simulink model "On_off_1_pumpstation"  (R2022b)
settings: Solver=VariableStepAuto  StartTime=0.0  StopTime=inf  RelTol=1e-3
libraries: modbusMatLib x24, realtime_pacer_lib x1
(part 1 of 2)
settings Model: Creator=pppc  LastModifiedBy=pppc
settings SolverCC: AlgebraicLoopSolver=TrustRegion
settings DebuggingCC: UnconnectedInputMsg=warning  UnconnectedOutputMsg=warning  UnconnectedLineMsg=warning  SFMachineParentedDataDiag=warning
settings ModelReferenceCC: EnableRefExpFcnMdlSchedulingChecks=on
settings RTWCC: DLArmComputeVersion=19.05

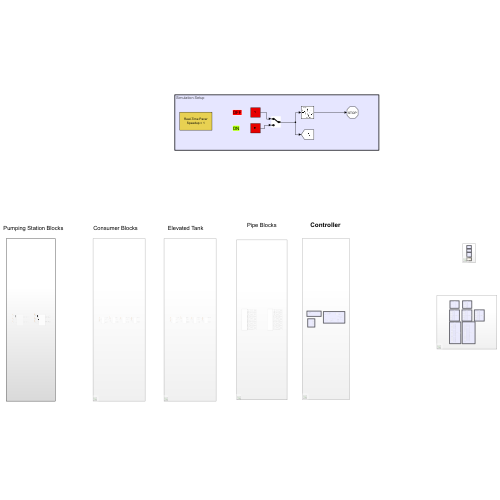
[thumbnail: Simulink's stored preview of the top-level diagram]
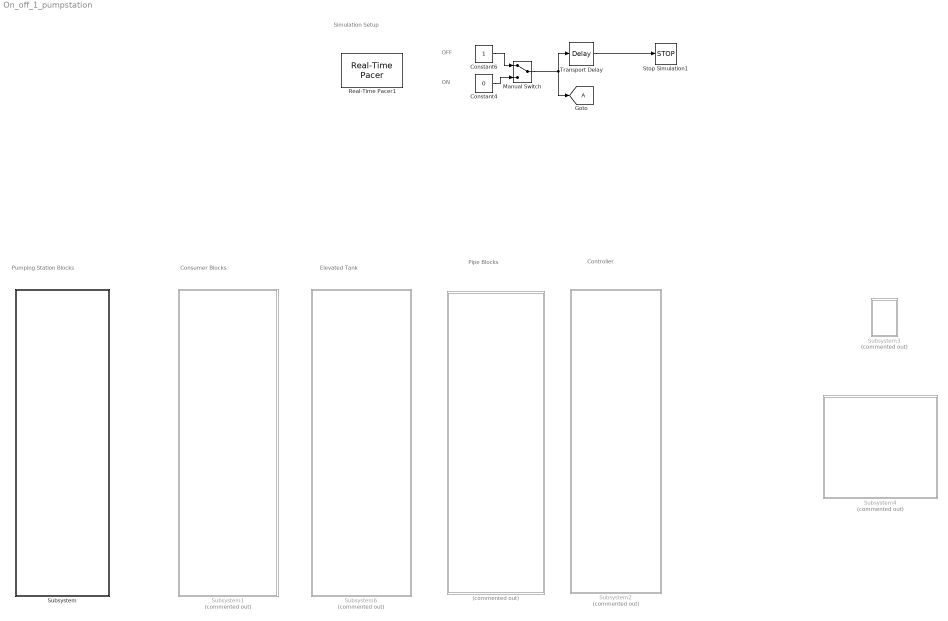
== system On_off_1_pumpstation ==
  note: Controller
  note: Pumping Station Blocks
  note: OFF
  note: ON
  note: Simulation Setup
  note: Consumer Blocks
  note: Pipe Blocks
  note: Elevated Tank
  " " : Subsystem  Commented=on
  Constant4 : Constant  Value=0
  Constant6 : Constant
  Goto : Goto  TagVisibility=global
  Manual Switch : ManualSwitch
  Real-Time Pacer1 : realtime_pacer_lib/Real-Time Pacer  simTimePerRealTime=1
  Stop Simulation1 : Stop
  Subsystem : Subsystem
  Subsystem1 : Subsystem  Commented=on
  Subsystem2 : Subsystem  Commented=on
  Subsystem3 : Subsystem  Commented=on
  Subsystem4 : Subsystem  Commented=on
  Subsystem6 : Subsystem  Commented=on
  Transport Delay : TransportDelay  DelayTime=2
  wires:
  Constant4/1 -> Manual Switch/2
  Transport Delay/1 -> Stop Simulation1/1
  Constant6/1 -> Manual Switch/1
  Manual Switch/1 -> Goto/1, Transport Delay/1

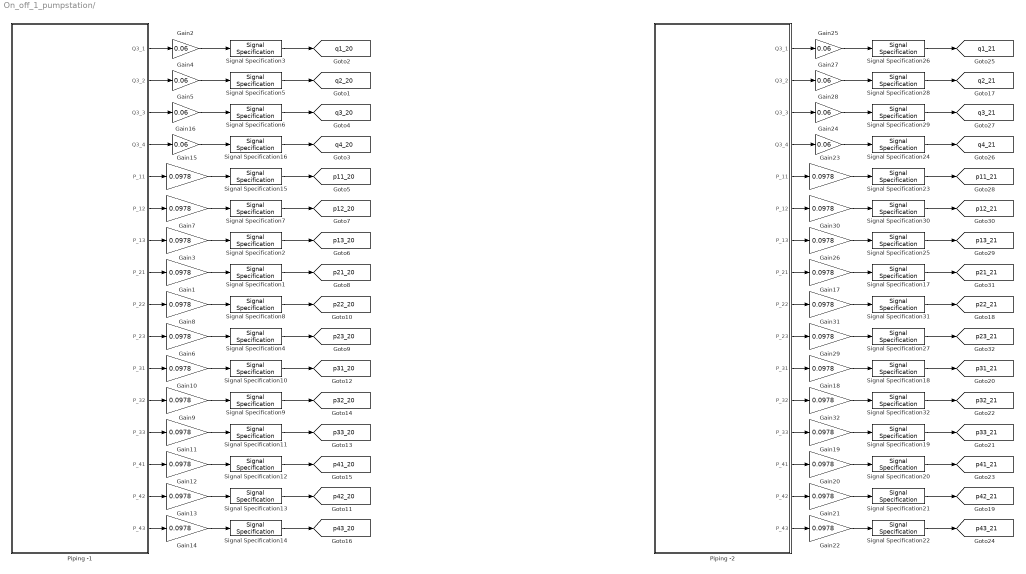
== system On_off_1_pumpstation/  ==
  Gain{1,3,6..15,17..23,26,29..32} (24 alike) : Gain  Gain=0.0978
  Gain{2,4..5,16,24..25,27..28} (8 alike) : Gain  Gain=0.06
  Piping -1 : Subsystem
  Piping -2 : Subsystem
  Signal Specification{1..2,4,7..15,17..23,25,27,30..32} (24 alike) : SignalSpecification  Unit=bar
  Signal Specification{3,5..6,16,24,26,28..29} (8 alike) : SignalSpecification  Unit=m^3/hr
  tag scope: p11_20=global, p11_21=global, p12_20=global, p12_21=global, p13_20=global, p13_21=global, p21_20=global, p21_21=global, p22_20=global, p22_21=global, p23_20=global, p23_21=global, p31_20=global, p31_21=global, p32_20=global, p32_21=global, p33_20=global, p33_21=global, p41_20=global, p41_21=global, p42_20=global, p42_21=global, p43_20=global, p43_21=global, q1_20=global, q1_21=global, q2_20=global, q2_21=global, q3_20=global, q3_21=global, q4_20=global, q4_21=global
  wires:
  Gain8/1 -> Signal Specification8/1
  Piping -1/6(P_12) -> Gain7/1
  Gain5/1 -> Signal Specification6/1
  Gain9/1 -> Signal Specification9/1
  Piping -1/12(P_32) -> Gain9/1
  Piping -1/9(P_22) -> Gain8/1
  Piping -1/3(Q3_3) -> Gain5/1
  Piping -1/2(Q3_2) -> Gain4/1
  Gain7/1 -> Signal Specification7/1
  Gain4/1 -> Signal Specification5/1
  Gain16/1 -> Signal Specification16/1
  Piping -1/4(Q3_4) -> Gain16/1
  Piping -1/1(Q3_1) -> Gain2/1
  Piping -1/8(P_21) -> Gain1/1
  Gain1/1 -> Signal Specification1/1
  Gain2/1 -> Signal Specification3/1
  Gain3/1 -> Signal Specification2/1
  Piping -1/7(P_13) -> Gain3/1
  Piping -1/10(P_23) -> Gain6/1
  Gain6/1 -> Signal Specification4/1
  Gain10/1 -> Signal Specification10/1
  Piping -1/11(P_31) -> Gain10/1
  Gain11/1 -> Signal Specification11/1
  Gain12/1 -> Signal Specification12/1
  Piping -1/13(P_33) -> Gain11/1
  Piping -1/14(P_41) -> Gain12/1
  Gain13/1 -> Signal Specification13/1
  Piping -1/15(P_42) -> Gain13/1
  Gain14/1 -> Signal Specification14/1
  Piping -1/16(P_43) -> Gain14/1
  Gain15/1 -> Signal Specification15/1
  Piping -1/5(P_11) -> Gain15/1
  Gain29/1 -> Signal Specification27/1
  Gain26/1 -> Signal Specification25/1
  Gain21/1 -> Signal Specification21/1
  Gain23/1 -> Signal Specification23/1
  Gain31/1 -> Signal Specification31/1
  Piping -2/15(P_42) -> Gain21/1
  Piping -2/5(P_11) -> Gain23/1
  Piping -2/16(P_43) -> Gain22/1
  Gain27/1 -> Signal Specification28/1
  Gain20/1 -> Signal Specification20/1
  Gain19/1 -> Signal Specification19/1
  Piping -2/14(P_41) -> Gain20/1
  Piping -2/13(P_33) -> Gain19/1
  Piping -2/12(P_32) -> Gain32/1
  Piping -2/6(P_12) -> Gain30/1
  Gain17/1 -> Signal Specification17/1
  Gain30/1 -> Signal Specification30/1
  Piping -2/3(Q3_3) -> Gain28/1
  Piping -2/7(P_13) -> Gain26/1
  Gain18/1 -> Signal Specification18/1
  Gain25/1 -> Signal Specification26/1
  Piping -2/4(Q3_4) -> Gain24/1
  Gain24/1 -> Signal Specification24/1
  Piping -2/8(P_21) -> Gain17/1
  Piping -2/1(Q3_1) -> Gain25/1
  Piping -2/11(P_31) -> Gain18/1
  Piping -2/9(P_22) -> Gain31/1
  Piping -2/10(P_23) -> Gain29/1
  Gain32/1 -> Signal Specification32/1
  Gain28/1 -> Signal Specification29/1
  Piping -2/2(Q3_2) -> Gain27/1
  Gain22/1 -> Signal Specification22/1
  Signal Specification3/1 -> [q1_20]
  Signal Specification5/1 -> [q2_20]
  Signal Specification6/1 -> [q3_20]
  Signal Specification16/1 -> [q4_20]
  Signal Specification2/1 -> [p13_20]
  Signal Specification15/1 -> [p11_20]
  Signal Specification7/1 -> [p12_20]
  Signal Specification8/1 -> [p22_20]
  Signal Specification4/1 -> [p23_20]
  Signal Specification1/1 -> [p21_20]
  Signal Specification13/1 -> [p42_20]
  Signal Specification12/1 -> [p41_20]
  Signal Specification14/1 -> [p43_20]
  Signal Specification9/1 -> [p32_20]
  Signal Specification11/1 -> [p33_20]
  Signal Specification10/1 -> [p31_20]
  Signal Specification32/1 -> [p32_21]
  Signal Specification26/1 -> [q1_21]
  Signal Specification21/1 -> [p42_21]
  Signal Specification19/1 -> [p33_21]
  Signal Specification20/1 -> [p41_21]
  Signal Specification18/1 -> [p31_21]
  Signal Specification27/1 -> [p23_21]
  Signal Specification31/1 -> [p22_21]
  Signal Specification24/1 -> [q4_21]
  Signal Specification30/1 -> [p12_21]
  Signal Specification23/1 -> [p11_21]
  Signal Specification28/1 -> [q2_21]
  Signal Specification29/1 -> [q3_21]
  Signal Specification17/1 -> [p21_21]
  Signal Specification22/1 -> [p43_21]
  Signal Specification25/1 -> [p13_21]

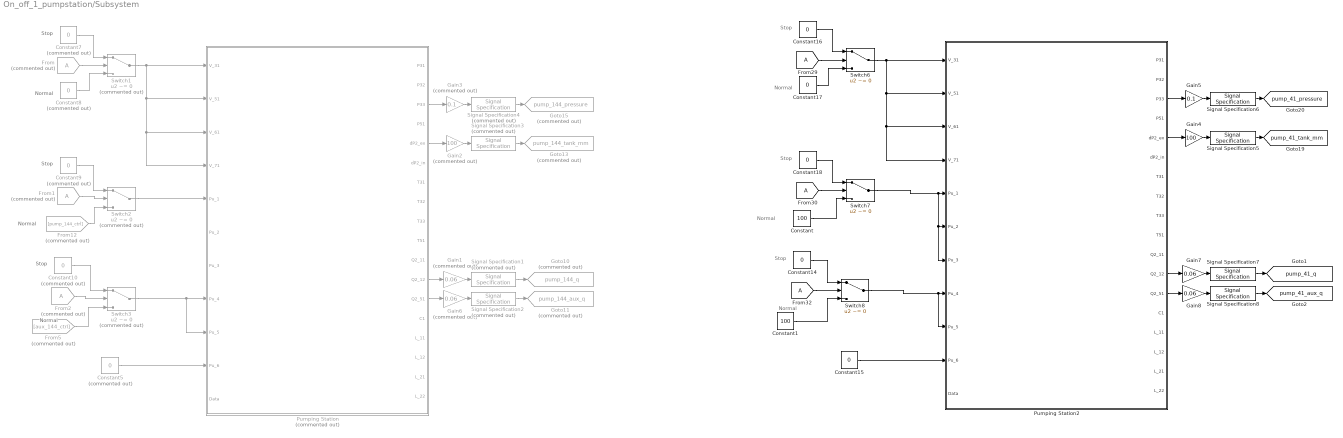
== system On_off_1_pumpstation/Subsystem ==
  note: Stop
  note: Normal
  note: Stop
  note: Normal
  note: Normal
  note: Stop
  note: Normal
  note: Stop
  note: Stop
  note: Normal
  note: Normal
  note: Stop
  Constant : Constant  Value=100
  Constant1 : Constant  Value=100
  Constant{5,7..10} (5 alike) : Constant  Commented=on  Value=0
  Constant{14..18} (5 alike) : Constant  Value=0
  From : From  Commented=on  TagVisibility=global
  From1 : From  Commented=on  TagVisibility=global
  From12 : From  Commented=on  GotoTag=pump_144_ctrl  TagVisibility=global
  From2 : From  Commented=on  TagVisibility=global
  From29 : From  TagVisibility=global
  From30 : From  TagVisibility=global
  From32 : From  TagVisibility=global
  From5 : From  Commented=on  GotoTag=aux_144_ctrl  TagVisibility=global
  Gain1 : Gain  Commented=on  Gain=0.06
  Gain2 : Gain  Commented=on  Gain=100
  Gain3 : Gain  Commented=on  Gain=0.1
  Gain4 : Gain  Gain=100
  Gain5 : Gain  Gain=0.1
  Gain6 : Gain  Commented=on  Gain=0.06
  Gain7 : Gain  Gain=0.06
  Gain8 : Gain  Gain=0.06
  Goto10 : Goto  Commented=on  GotoTag=pump_144_q  TagVisibility=global
  Goto11 : Goto  Commented=on  GotoTag=pump_144_aux_q  TagVisibility=global
  Goto13 : Goto  Commented=on  GotoTag=pump_144_tank_mm  TagVisibility=global
  Goto15 : Goto  Commented=on  GotoTag=pump_144_pressure  TagVisibility=global
  Pumping Station : Subsystem  Commented=on
  Pumping Station2 : Subsystem
  Signal Specification1 : SignalSpecification  Commented=on  Unit=m^3/hr
  Signal Specification2 : SignalSpecification  Commented=on  Unit=m^3/hr
  Signal Specification3 : SignalSpecification  Commented=on  Unit=mm
  Signal Specification4 : SignalSpecification  Commented=on  Unit=bar
  Signal Specification5 : SignalSpecification  Unit=mm
  Signal Specification6 : SignalSpecification  Unit=bar
  Signal Specification7 : SignalSpecification  Unit=m^3/hr
  Signal Specification8 : SignalSpecification  Unit=m^3/hr
  Switch1 : Switch  Commented=on  Criteria=u2 ~= 0  SaturateOnIntegerOverflow=off  InputSameDT=off
  Switch2 : Switch  Commented=on  Criteria=u2 ~= 0  SaturateOnIntegerOverflow=off  InputSameDT=off
  Switch3 : Switch  Commented=on  Criteria=u2 ~= 0  SaturateOnIntegerOverflow=off  InputSameDT=off
  Switch6 : Switch  Criteria=u2 ~= 0  SaturateOnIntegerOverflow=off  InputSameDT=off
  Switch7 : Switch  Criteria=u2 ~= 0  SaturateOnIntegerOverflow=off  InputSameDT=off
  Switch8 : Switch  Criteria=u2 ~= 0  SaturateOnIntegerOverflow=off  InputSameDT=off
  tag scope: pump_41_aux_q=global, pump_41_pressure=global, pump_41_q=global, pump_41_tank_mm=global
  wires:
  From2/1 -> Switch3/2
  Gain3/1 -> Signal Specification4/1
  Constant1/1 -> Switch8/3
  Pumping Station/3(P33) -> Gain3/1
  Signal Specification6/1 -> [pump_41_pressure]
  Pumping Station2/5(dP2_ex) -> Gain4/1
  From12/1 -> Switch2/3
  Constant5/1 -> Pumping Station/10(Pu_6)
  From1/1 -> Switch2/2
  Switch1/1 -> Pumping Station/4(V_71), Pumping Station/3(V_61), Pumping Station/2(V_51), Pumping Station/1(V_31)
  Switch6/1 -> Pumping Station2/4(V_71), Pumping Station2/3(V_61), Pumping Station2/2(V_51), Pumping Station2/1(V_31)
  Pumping Station/5(dP2_ex) -> Gain2/1
  Constant9/1 -> Switch2/1
  Constant/1 -> Switch7/3
  Signal Specification2/1 -> Goto11/1
  From32/1 -> Switch8/2
  Signal Specification5/1 -> [pump_41_tank_mm]
  Signal Specification3/1 -> Goto13/1
  From5/1 -> Switch3/3
  Signal Specification1/1 -> Goto10/1
  Constant8/1 -> Switch1/3
  From29/1 -> Switch6/2
  Constant7/1 -> Switch1/1
  Signal Specification4/1 -> Goto15/1
  Constant17/1 -> Switch6/3
  Constant16/1 -> Switch6/1
  Constant10/1 -> Switch3/1
  Switch2/1 -> Pumping Station/5(Pu_1)
  Switch7/1 -> Pumping Station2/7(Pu_3), Pumping Station2/6(Pu_2), Pumping Station2/5(Pu_1)
  Switch8/1 -> Pumping Station2/9(Pu_5), Pumping Station2/8(Pu_4)
  Constant18/1 -> Switch7/1
  From30/1 -> Switch7/2
  Gain5/1 -> Signal Specification6/1
  Gain2/1 -> Signal Specification3/1
  Gain4/1 -> Signal Specification5/1
  From/1 -> Switch1/2
  Pumping Station2/3(P33) -> Gain5/1
  Constant14/1 -> Switch8/1
  Switch3/1 -> Pumping Station/9(Pu_5), Pumping Station/8(Pu_4)
  Constant15/1 -> Pumping Station2/10(Pu_6)
  Gain1/1 -> Signal Specification1/1
  Pumping Station/12(Q2_12) -> Gain1/1
  Pumping Station/13(Q2_51) -> Gain6/1
  Gain6/1 -> Signal Specification2/1
  Gain8/1 -> Signal Specification8/1
  Signal Specification8/1 -> [pump_41_aux_q]
  Pumping Station2/13(Q2_51) -> Gain8/1
  Pumping Station2/12(Q2_12) -> Gain7/1
  Gain7/1 -> Signal Specification7/1
  Signal Specification7/1 -> [pump_41_q]

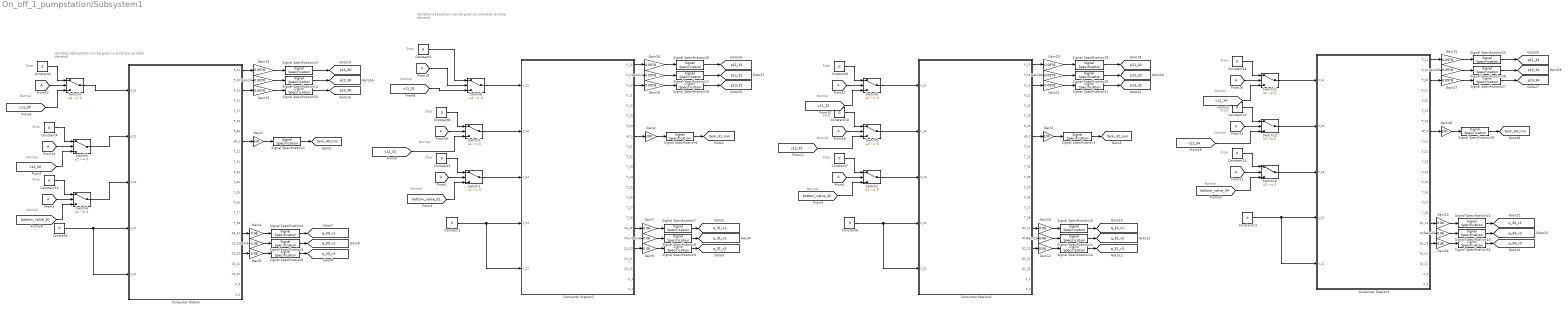
== system On_off_1_pumpstation/Subsystem1 ==
  note: Normal
  note: Variable load pattern can be
      | given to simulate variable demand
  note: Normal
  note: Stop
  note: Normal
  note: Variable load pattern can be
      | given to simulate variable demand
  note: Stop
  note: Normal
  note: Normal
  note: Stop
  note: Stop
  note: Normal
  note: Normal
  note: Stop
  note: Stop
  note: Stop
  note: Stop
  note: Stop
  note: Normal
  note: Normal
  note: Stop
  note: Normal
  note: Stop
  note: Stop
  note: Normal
  note: Normal
  Constant{,1..15} (16 alike) : Constant  Value=0
  Consumer Station : Subsystem
  Consumer Station1 : Subsystem
  Consumer Station2 : Subsystem
  Consumer Station3 : Subsystem
  From{1..3,13..18,20..22} (12 alike) : From  TagVisibility=global
  Gain{1..3,28} (4 alike) : Gain  Gain=100
  Gain{4..12,22..24} (12 alike) : Gain  Gain=0.06
  Gain{13..21,25..27} (12 alike) : Gain  Gain=0.0978
  Signal Specification{1..3,28} (4 alike) : SignalSpecification  Unit=mm
  Signal Specification{4..12,22..24} (12 alike) : SignalSpecification  Unit=m^3/hr
  Signal Specification{13..21,25..27} (12 alike) : SignalSpecification  Unit=bar
  Switch{1..12} (12 alike) : Switch  Criteria=u2 ~= 0  SaturateOnIntegerOverflow=off  InputSameDT=off
  tag scope: p11_30=global, p11_31=global, p11_32=global, p11_34=global, p12_30=global, p12_31=global, p12_32=global, p12_34=global, p13_30=global, p13_31=global, p13_32=global, p13_34=global, q_30_v1=global, q_30_v2=global, q_30_v3=global, q_31_v1=global, q_31_v2=global, q_31_v3=global, q_32_v1=global, q_32_v2=global, q_32_v3=global, q_34_v1=global, q_34_v2=global, q_34_v3=global, tank_30_mm=global, tank_31_mm=global, tank_32_mm=global, tank_34_mm=global
  wires:
  [v12_32] -> Switch9/3
  Consumer Station2/1(P_11) -> Gain19/1
  Consumer Station2/19(Q1_13) -> Gain12/1
  [bottom_valve_32] -> Switch2/3
  Gain16/1 -> Signal Specification16/1
  Consumer Station1/1(P_11) -> Gain16/1
  Signal Specification16/1 -> [p11_31]
  Gain14/1 -> Signal Specification14/1
  Gain17/1 -> Signal Specification17/1
  Gain12/1 -> Signal Specification12/1
  Signal Specification15/1 -> [p13_30]
  Consumer Station1/3(P_13) -> Gain18/1
  Signal Specification14/1 -> [p12_30]
  Switch1/1 -> Consumer Station1/3(V_13)
  Gain20/1 -> Signal Specification20/1
  Signal Specification18/1 -> [p13_31]
  Consumer Station1/2(P_12) -> Gain17/1
  Gain7/1 -> Signal Specification7/1
  Gain9/1 -> Signal Specification9/1
  Signal Specification13/1 -> [p11_30]
  Signal Specification11/1 -> [q_32_v2]
  Constant7/1 -> Switch2/1
  Signal Specification10/1 -> [q_32_v1]
  Gain8/1 -> Signal Specification8/1
  Consumer Station2/17(Q1_11) -> Gain10/1
  Gain13/1 -> Signal Specification13/1
  Signal Specification8/1 -> [q_31_v2]
  Consumer Station1/19(Q1_13) -> Gain9/1
  Consumer Station2/18(Q1_12) -> Gain11/1
  Consumer Station/2(P_12) -> Gain14/1
  Consumer Station/1(P_11) -> Gain13/1
  Signal Specification5/1 -> [q_30_v2]
  Constant3/1 -> Switch1/1
  Gain5/1 -> Signal Specification5/1
  From2/1 -> Switch2/2
  Consumer Station2/8(dP_2) -> Gain3/1
  Gain4/1 -> Signal Specification4/1
  [bottom_valve_31] -> Switch1/3
  Consumer Station1/18(Q1_12) -> Gain8/1
  Gain3/1 -> Signal Specification3/1
  Signal Specification3/1 -> [tank_32_mm]
  Signal Specification7/1 -> [q_31_v1]
  Switch2/1 -> Consumer Station2/3(V_13)
  Consumer Station1/8(dP_2) -> Gain2/1
  [bottom_valve_30] -> Switch4/3
  Constant1/1 -> Consumer Station1/5(V_22), Consumer Station1/4(V_21)
  Constant11/1 -> Switch4/1
  Signal Specification4/1 -> [q_30_v1]
  Signal Specification19/1 -> [p11_32]
  Switch4/1 -> Consumer Station/3(V_13)
  Consumer Station1/17(Q1_11) -> Gain7/1
  Gain18/1 -> Signal Specification18/1
  Consumer Station/18(Q1_12) -> Gain5/1
  From17/1 -> Switch8/2
  Switch9/1 -> Consumer Station2/2(V_12)
  From13/1 -> Switch3/2
  [v11_32] -> Switch8/3
  Gain6/1 -> Signal Specification6/1
  Signal Specification12/1 -> [q_32_v3]
  Gain19/1 -> Signal Specification19/1
  [v11_31] -> Switch6/3
  Gain15/1 -> Signal Specification15/1
  Switch6/1 -> Consumer Station1/1(V_11)
  From15/1 -> Switch6/2
  Consumer Station/8(dP_2) -> Gain1/1
  Consumer Station/17(Q1_11) -> Gain4/1
  From18/1 -> Switch9/2
  Constant10/1 -> Switch9/1
  Constant5/1 -> Switch6/1
  Switch3/1 -> Consumer Station/1(V_11)
  Constant9/1 -> Switch8/1
  Switch8/1 -> Consumer Station2/1(V_11)
  Gain11/1 -> Signal Specification11/1
  Consumer Station2/3(P_13) -> Gain21/1
  Constant8/1 -> Switch7/1
  Switch7/1 -> Consumer Station1/2(V_12)
  [v12_31] -> Switch7/3
  From16/1 -> Switch7/2
  Signal Specification6/1 -> [q_30_v3]
  [v11_30] -> Switch3/3
  Signal Specification1/1 -> [tank_30_mm]
  Switch5/1 -> Consumer Station/2(V_12)
  [v12_30] -> Switch5/3
  Signal Specification2/1 -> [tank_31_mm]
  Signal Specification17/1 -> [p12_31]
  Gain2/1 -> Signal Specification2/1
  Consumer Station2/2(P_12) -> Gain20/1
  Gain1/1 -> Signal Specification1/1
  From3/1 -> Switch4/2
  Constant/1 -> Consumer Station/5(V_22), Consumer Station/4(V_21)
  Gain21/1 -> Signal Specification21/1
  Constant4/1 -> Switch5/1
  Consumer Station/3(P_13) -> Gain15/1
  Consumer Station/19(Q1_13) -> Gain6/1
  Constant6/1 -> Consumer Station2/5(V_22), Consumer Station2/4(V_21)
  Constant2/1 -> Switch3/1
  Signal Specification20/1 -> [p12_32]
  From14/1 -> Switch5/2
  From1/1 -> Switch1/2
  Signal Specification21/1 -> [p13_32]
  Gain10/1 -> Signal Specification10/1
  Signal Specification9/1 -> [q_31_v3]
  Signal Specification22/1 -> [q_34_v1]
  [v12_34] -> Switch12/3
  Gain24/1 -> Signal Specification24/1
  Consumer Station3/17(Q1_11) -> Gain22/1
  From22/1 -> Switch10/2
  Consumer Station3/1(P_11) -> Gain25/1
  Signal Specification26/1 -> [p12_34]
  [bottom_valve_34] -> Switch10/3
  Signal Specification27/1 -> [p13_34]
  Gain25/1 -> Signal Specification25/1
  Consumer Station3/2(P_12) -> Gain26/1
  Signal Specification28/1 -> [tank_34_mm]
  Gain22/1 -> Signal Specification22/1
  Gain27/1 -> Signal Specification27/1
  Signal Specification23/1 -> [q_34_v2]
  Constant15/1 -> Switch11/1
  Consumer Station3/18(Q1_12) -> Gain23/1
  Constant13/1 -> Consumer Station3/5(V_22), Consumer Station3/4(V_21)
  Constant12/1 -> Switch12/1
  Gain23/1 -> Signal Specification23/1
  Gain26/1 -> Signal Specification26/1
  Switch11/1 -> Consumer Station3/1(V_11)
  Switch12/1 -> Consumer Station3/2(V_12)
  Consumer Station3/3(P_13) -> Gain27/1
  [v11_34] -> Switch11/3
  Constant14/1 -> Switch10/1
  Consumer Station3/8(dP_2) -> Gain28/1
  Signal Specification24/1 -> [q_34_v3]
  Switch10/1 -> Consumer Station3/3(V_13)
  From21/1 -> Switch12/2
  Signal Specification25/1 -> [p11_34]
  From20/1 -> Switch11/2
  Gain28/1 -> Signal Specification28/1
  Consumer Station3/19(Q1_13) -> Gain24/1

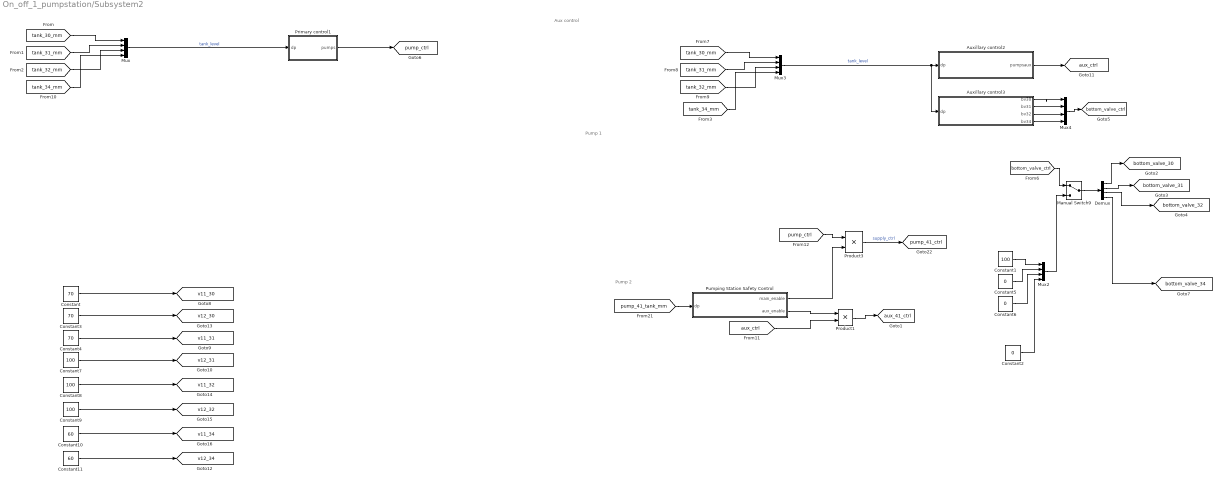
== system On_off_1_pumpstation/Subsystem2 ==
  note: Pump 1
  note: Aux control
  note: Pump 2
  Auxillary control2 : MATLAB Function  TreatAsAtomicUnit=on
  Auxillary control3 : MATLAB Function  TreatAsAtomicUnit=on
  Constant : Constant  Value=70
  Constant{1,7..9} (4 alike) : Constant  Value=100
  Constant10 : Constant  Value=60
  Constant11 : Constant  Value=60
  Constant2 : Constant  Value=0
  Constant3 : Constant  Value=70
  Constant4 : Constant  Value=70
  Constant5 : Constant  Value=0
  Constant6 : Constant  Value=0
  Demux : Demux
  Manual Switch9 : ManualSwitch
  Mux{,2..4} (4 alike) : Mux
  Primary control1 : MATLAB Function  TreatAsAtomicUnit=on
  Product1 : Product
  Product3 : Product
  Pumping Station Safety Control : MATLAB Function  TreatAsAtomicUnit=on
  tag scope: aux_41_ctrl=global, aux_ctrl=global, bottom_valve_30=global, bottom_valve_31=global, bottom_valve_32=global, bottom_valve_34=global, bottom_valve_ctrl=global, pump_41_ctrl=global, pump_ctrl=global, v11_30=global, v11_31=global, v11_32=global, v11_34=global, v12_30=global, v12_31=global, v12_32=global, v12_34=global
  wires:
  Primary control1/1(pumps) -> [pump_ctrl]
  Mux/1 -> Primary control1/1(dp)  "tank_level"
  [tank_30_mm] -> Mux/1
  [tank_31_mm] -> Mux/2
  [tank_32_mm] -> Mux/3
  [tank_34_mm] -> Mux/4
  Mux4/1 -> [bottom_valve_ctrl]
  Constant1/1 -> Mux2/1
  Mux2/1 -> Manual Switch9/2
  Auxillary control3/1(bv30) -> Mux4/1
  Constant5/1 -> Mux2/2
  Manual Switch9/1 -> Demux/1
  Auxillary control3/2(bv31) -> Mux4/2
  [tank_32_mm] -> Mux3/3
  [bottom_valve_ctrl] -> Manual Switch9/1
  Demux/2 -> [bottom_valve_31]
  Auxillary control2/1(pumpsaux) -> [aux_ctrl]
  Demux/1 -> [bottom_valve_30]
  Pumping Station Safety Control/2(aux_enable) -> Product1/1
  [pump_41_tank_mm] -> Pumping Station Safety Control/1(dp)
  [tank_30_mm] -> Mux3/1
  [tank_31_mm] -> Mux3/2
  Mux3/1 -> Auxillary control3/1(dp), Auxillary control2/1(dp)  "tank_level"
  Constant6/1 -> Mux2/3
  [aux_ctrl] -> Product1/2
  Demux/3 -> [bottom_valve_32]
  Product1/1 -> [aux_41_ctrl]
  Auxillary control3/3(bv32) -> Mux4/3
  [tank_34_mm] -> Mux3/4
  Demux/4 -> [bottom_valve_34]
  [pump_ctrl] -> Product3/1
  Product3/1 -> [pump_41_ctrl]  "supply_ctrl"
  Pumping Station Safety Control/1(main_enable) -> Product3/2
  Constant2/1 -> Mux2/4
  Auxillary control3/4(bv34) -> Mux4/4
  Constant/1 -> [v11_30]
  Constant3/1 -> [v12_30]
  Constant4/1 -> [v11_31]
  Constant7/1 -> [v12_31]
  Constant8/1 -> [v11_32]
  Constant9/1 -> [v12_32]
  Constant10/1 -> [v11_34]
  Constant11/1 -> [v12_34]

== system On_off_1_pumpstation/Subsystem3 ==
  note: TO WORKSPACE
  note: Pumping scopes
  note: Demand scopes
  note: Reservoir scopes
  Consumer tank : Scope  Commented=on  NumInputPorts=3
  Elevated reservoir : Scope  Commented=on  NumInputPorts=2
  Flow of auxillary pump : Scope  Commented=on  NumInputPorts=2
  From10 : From  Commented=on  GotoTag=resvr_tank_mm
  From11 : From  Commented=on  GotoTag=resvr_tank_q
  From13 : From  Commented=on  GotoTag=pump_1_ctrl  TagVisibility=global
  From15 : From  Commented=on  GotoTag=d1_q
  From16 : From  Commented=on  GotoTag=d2_q
  From17 : From  Commented=on  GotoTag=dem_tank_out_q
  From18 : From  Commented=on  GotoTag=pump_1_q  TagVisibility=global
  From19 : From  Commented=on  GotoTag=pump_aux_q  TagVisibility=global
  From20 : From  Commented=on  GotoTag=pump_1_q_mag
  From22 : From  Commented=on  GotoTag=pump_tank_mm  TagVisibility=global
  From23 : From  Commented=on  GotoTag=pipe_3_q_mag
  From24 : From  Commented=on  GotoTag=supply_pressure  TagVisibility=global
  From25 : From  Commented=on  GotoTag=pump_1_q_mag
  From26 : From  Commented=on  GotoTag=pump_1_ctrl  TagVisibility=global
  From6 : From  Commented=on  GotoTag=aux_ctrl
  From8 : From  Commented=on  GotoTag=dem_tank_mm
  Level of pump external tank : Scope  Commented=on  NumInputPorts=4
  Mux1 : Mux  Commented=on  Inputs=2
  Mux2 : Mux  Commented=on  Inputs=2
  Pipe flow : Scope  Commented=on
  To Workspace : ToWorkspace  Commented=on  VariableName=pump_control  SampleTime=-1
      settings: Save2DSignal=2-D array (concatenate along first dimension)
  To Workspace1 : ToWorkspace  Commented=on  VariableName=flow  SampleTime=-1
      settings: Save2DSignal=2-D array (concatenate along first dimension)
  wires:
  From15/1 -> Mux1/1
  From22/1 -> Level of pump external tank/1
  From11/1 -> Elevated reservoir/2
  From8/1 -> Consumer tank/1
  Mux1/1 -> Consumer tank/3
  From16/1 -> Mux1/2
  From18/1 -> Mux2/1
  From24/1 -> Level of pump external tank/2
  From20/1 -> Mux2/2
  From23/1 -> Pipe flow/1
  From26/1 -> To Workspace/1
  From10/1 -> Elevated reservoir/1
  From13/1 -> Level of pump external tank/4
  From19/1 -> Flow of auxillary pump/1
  From17/1 -> Consumer tank/2
  From6/1 -> Flow of auxillary pump/2
  Mux2/1 -> Level of pump external tank/3
  From25/1 -> To Workspace1/1

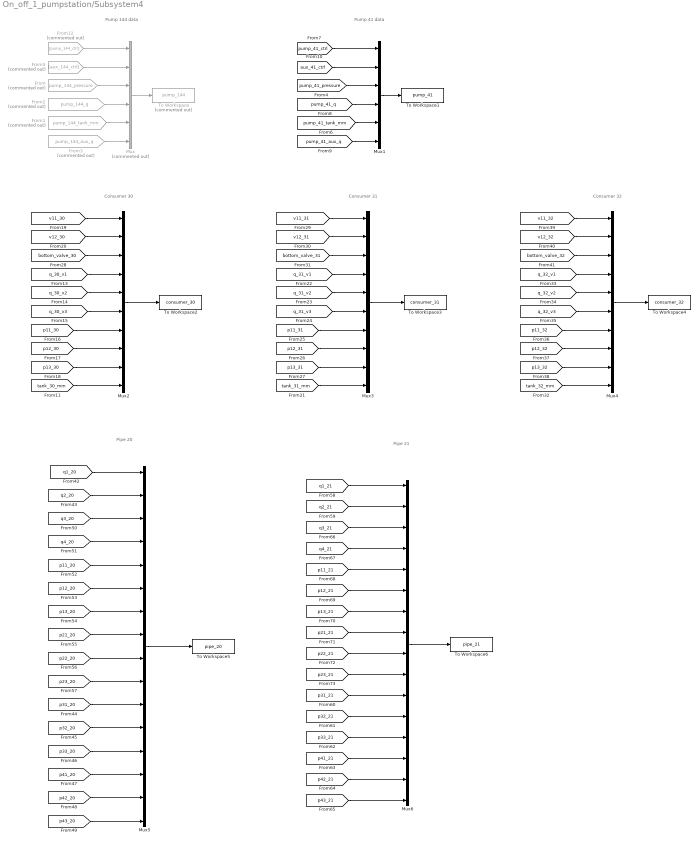
== system On_off_1_pumpstation/Subsystem4 ==
  note: Pipe 21
  note: Pipe 20
  note: Consumer 30
  note: Pump 144 data
  note: Pump 41 data
  note: Consumer 31
  note: Consumer 32
  From : From  Commented=on  GotoTag=pump_144_pressure  TagVisibility=global
  From1 : From  Commented=on  GotoTag=pump_144_tank_mm  TagVisibility=global
  From12 : From  Commented=on  GotoTag=pump_144_ctrl  TagVisibility=global
  From2 : From  Commented=on  GotoTag=pump_144_q  TagVisibility=global
  From3 : From  Commented=on  GotoTag=pump_144_aux_q  TagVisibility=global
  From5 : From  Commented=on  GotoTag=aux_144_ctrl  TagVisibility=global
  Mux : Mux  Commented=on  Inputs=6
  Mux1 : Mux  Inputs=6
  Mux2 : Mux  Inputs=10
  Mux3 : Mux  Inputs=10
  Mux4 : Mux  Inputs=10
  Mux5 : Mux  Inputs=16
  Mux6 : Mux  Inputs=16
  To Workspace : ToWorkspace  Commented=on  VariableName=pump_144  SaveFormat=Structure With Time  SampleTime=1
      settings: Save2DSignal=2-D array (concatenate along first dimension)
  To Workspace1 : ToWorkspace  VariableName=pump_41  SaveFormat=Structure With Time  SampleTime=1
  To Workspace2 : ToWorkspace  VariableName=consumer_30  SaveFormat=Structure With Time  SampleTime=1
  To Workspace3 : ToWorkspace  VariableName=consumer_31  SaveFormat=Structure With Time  SampleTime=1
  To Workspace4 : ToWorkspace  VariableName=consumer_32  SaveFormat=Structure With Time  SampleTime=1
  To Workspace5 : ToWorkspace  VariableName=pipe_20  SaveFormat=Structure With Time  SampleTime=1
  To Workspace6 : ToWorkspace  VariableName=pipe_21  SaveFormat=Structure With Time  SampleTime=1
  wires:
  From12/1 -> Mux/1
  From5/1 -> Mux/2
  From/1 -> Mux/3
  From2/1 -> Mux/4
  From1/1 -> Mux/5
  From3/1 -> Mux/6
  Mux/1 -> To Workspace/1
  [pump_41_tank_mm] -> Mux1/5
  [aux_41_ctrl] -> Mux1/2
  [pump_41_aux_q] -> Mux1/6
  [pump_41_pressure] -> Mux1/3
  [pump_41_ctrl] -> Mux1/1
  [pump_41_q] -> Mux1/4
  Mux1/1 -> To Workspace1/1
  [v11_30] -> Mux2/1
  [tank_30_mm] -> Mux2/10
  [p13_30] -> Mux2/9
  [p12_30] -> Mux2/8
  [p11_30] -> Mux2/7
  [q_30_v3] -> Mux2/6
  [q_30_v2] -> Mux2/5
  [q_30_v1] -> Mux2/4
  [bottom_valve_30] -> Mux2/3
  [v12_30] -> Mux2/2
  Mux2/1 -> To Workspace2/1
  [tank_31_mm] -> Mux3/10
  [p13_31] -> Mux3/9
  [q_31_v2] -> Mux3/5
  Mux3/1 -> To Workspace3/1
  [bottom_valve_31] -> Mux3/3
  [q_31_v1] -> Mux3/4
  [v11_31] -> Mux3/1
  [v12_31] -> Mux3/2
  [q_31_v3] -> Mux3/6
  [p11_31] -> Mux3/7
  [p12_31] -> Mux3/8
  [tank_32_mm] -> Mux4/10
  [p13_32] -> Mux4/9
  [q_32_v2] -> Mux4/5
  Mux4/1 -> To Workspace4/1
  [bottom_valve_32] -> Mux4/3
  [q_32_v1] -> Mux4/4
  [v11_32] -> Mux4/1
  [v12_32] -> Mux4/2
  [q_32_v3] -> Mux4/6
  [p11_32] -> Mux4/7
  [p12_32] -> Mux4/8
  [p43_20] -> Mux5/16
  [q1_20] -> Mux5/1
  [p42_20] -> Mux5/15
  [p41_20] -> Mux5/14
  [p33_20] -> Mux5/13
  [p32_20] -> Mux5/12
  [p31_20] -> Mux5/11
  [p23_20] -> Mux5/10
  [p22_20] -> Mux5/9
  [p21_20] -> Mux5/8
  [p13_20] -> Mux5/7
  [p12_20] -> Mux5/6
  [p11_20] -> Mux5/5
  [q4_20] -> Mux5/4
  [q3_20] -> Mux5/3
  [q2_20] -> Mux5/2
  Mux5/1 -> To Workspace5/1
  [q1_21] -> Mux6/1
  [p43_21] -> Mux6/16
  [p42_21] -> Mux6/15
  [p41_21] -> Mux6/14
  [p33_21] -> Mux6/13
  [p32_21] -> Mux6/12
  [p31_21] -> Mux6/11
  [p23_21] -> Mux6/10
  [p22_21] -> Mux6/9
  [p21_21] -> Mux6/8
  [p13_21] -> Mux6/7
  [p12_21] -> Mux6/6
  [p11_21] -> Mux6/5
  [q4_21] -> Mux6/4
  [q3_21] -> Mux6/3
  [q2_21] -> Mux6/2
  Mux6/1 -> To Workspace6/1

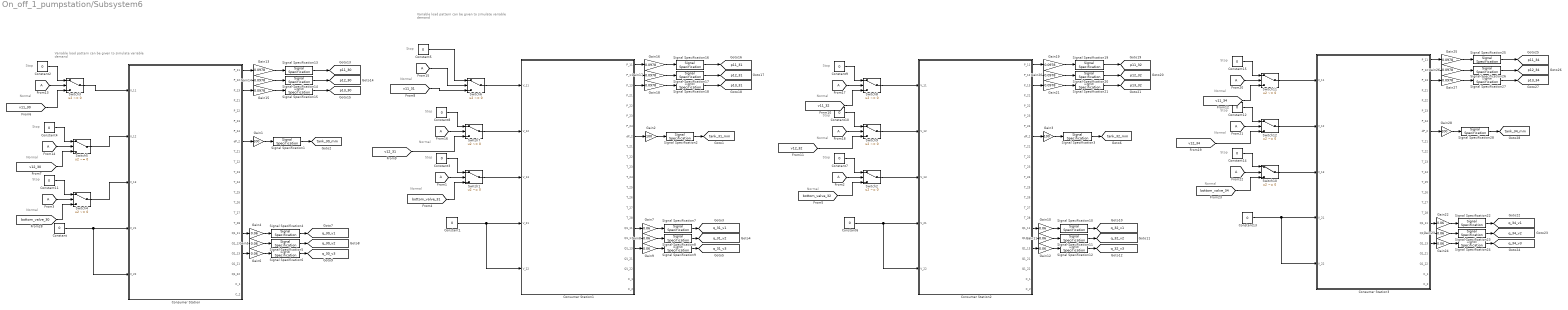
== system On_off_1_pumpstation/Subsystem6 ==
  note: Normal
  note: Variable load pattern can be
      | given to simulate variable demand
  note: Normal
  note: Stop
  note: Normal
  note: Variable load pattern can be
      | given to simulate variable demand
  note: Stop
  note: Normal
  note: Normal
  note: Stop
  note: Stop
  note: Normal
  note: Normal
  note: Stop
  note: Stop
  note: Stop
  note: Stop
  note: Stop
  note: Normal
  note: Normal
  note: Stop
  note: Normal
  note: Stop
  note: Stop
  note: Normal
  note: Normal
  Constant{,1..15} (16 alike) : Constant  Value=0
  Consumer Station : Subsystem
  Consumer Station1 : Subsystem
  Consumer Station2 : Subsystem
  Consumer Station3 : Subsystem
  From{1..3,13..18,20..22} (12 alike) : From  TagVisibility=global
  Gain{1..3,28} (4 alike) : Gain  Gain=100
  Gain{4..12,22..24} (12 alike) : Gain  Gain=0.06
  Gain{13..21,25..27} (12 alike) : Gain  Gain=0.0978
  Signal Specification{1..3,28} (4 alike) : SignalSpecification  Unit=mm
  Signal Specification{4..12,22..24} (12 alike) : SignalSpecification  Unit=m^3/hr
  Signal Specification{13..21,25..27} (12 alike) : SignalSpecification  Unit=bar
  Switch{1..12} (12 alike) : Switch  Criteria=u2 ~= 0  SaturateOnIntegerOverflow=off  InputSameDT=off
  tag scope: p11_30=global, p11_31=global, p11_32=global, p11_34=global, p12_30=global, p12_31=global, p12_32=global, p12_34=global, p13_30=global, p13_31=global, p13_32=global, p13_34=global, q_30_v1=global, q_30_v2=global, q_30_v3=global, q_31_v1=global, q_31_v2=global, q_31_v3=global, q_32_v1=global, q_32_v2=global, q_32_v3=global, q_34_v1=global, q_34_v2=global, q_34_v3=global, tank_30_mm=global, tank_31_mm=global, tank_32_mm=global, tank_34_mm=global
  wires:
  [v12_32] -> Switch9/3
  Consumer Station2/1(P_11) -> Gain19/1
  Consumer Station2/19(Q1_13) -> Gain12/1
  [bottom_valve_32] -> Switch2/3
  Gain16/1 -> Signal Specification16/1
  Consumer Station1/1(P_11) -> Gain16/1
  Signal Specification16/1 -> [p11_31]
  Gain14/1 -> Signal Specification14/1
  Gain17/1 -> Signal Specification17/1
  Gain12/1 -> Signal Specification12/1
  Signal Specification15/1 -> [p13_30]
  Consumer Station1/3(P_13) -> Gain18/1
  Signal Specification14/1 -> [p12_30]
  Switch1/1 -> Consumer Station1/3(V_13)
  Gain20/1 -> Signal Specification20/1
  Signal Specification18/1 -> [p13_31]
  Consumer Station1/2(P_12) -> Gain17/1
  Gain7/1 -> Signal Specification7/1
  Gain9/1 -> Signal Specification9/1
  Signal Specification13/1 -> [p11_30]
  Signal Specification11/1 -> [q_32_v2]
  Constant7/1 -> Switch2/1
  Signal Specification10/1 -> [q_32_v1]
  Gain8/1 -> Signal Specification8/1
  Consumer Station2/17(Q1_11) -> Gain10/1
  Gain13/1 -> Signal Specification13/1
  Signal Specification8/1 -> [q_31_v2]
  Consumer Station1/19(Q1_13) -> Gain9/1
  Consumer Station2/18(Q1_12) -> Gain11/1
  Consumer Station/2(P_12) -> Gain14/1
  Consumer Station/1(P_11) -> Gain13/1
  Signal Specification5/1 -> [q_30_v2]
  Constant3/1 -> Switch1/1
  Gain5/1 -> Signal Specification5/1
  From2/1 -> Switch2/2
  Consumer Station2/8(dP_2) -> Gain3/1
  Gain4/1 -> Signal Specification4/1
  [bottom_valve_31] -> Switch1/3
  Consumer Station1/18(Q1_12) -> Gain8/1
  Gain3/1 -> Signal Specification3/1
  Signal Specification3/1 -> [tank_32_mm]
  Signal Specification7/1 -> [q_31_v1]
  Switch2/1 -> Consumer Station2/3(V_13)
  Consumer Station1/8(dP_2) -> Gain2/1
  [bottom_valve_30] -> Switch4/3
  Constant1/1 -> Consumer Station1/5(V_22), Consumer Station1/4(V_21)
  Constant11/1 -> Switch4/1
  Signal Specification4/1 -> [q_30_v1]
  Signal Specification19/1 -> [p11_32]
  Switch4/1 -> Consumer Station/3(V_13)
  Consumer Station1/17(Q1_11) -> Gain7/1
  Gain18/1 -> Signal Specification18/1
  Consumer Station/18(Q1_12) -> Gain5/1
  From17/1 -> Switch8/2
  Switch9/1 -> Consumer Station2/2(V_12)
  From13/1 -> Switch3/2
  [v11_32] -> Switch8/3
  Gain6/1 -> Signal Specification6/1
  Signal Specification12/1 -> [q_32_v3]
  Gain19/1 -> Signal Specification19/1
  [v11_31] -> Switch6/3
  Gain15/1 -> Signal Specification15/1
  Switch6/1 -> Consumer Station1/1(V_11)
  From15/1 -> Switch6/2
  Consumer Station/8(dP_2) -> Gain1/1
  Consumer Station/17(Q1_11) -> Gain4/1
  From18/1 -> Switch9/2
  Constant10/1 -> Switch9/1
  Constant5/1 -> Switch6/1
  Switch3/1 -> Consumer Station/1(V_11)
  Constant9/1 -> Switch8/1
  Switch8/1 -> Consumer Station2/1(V_11)
  Gain11/1 -> Signal Specification11/1
  Consumer Station2/3(P_13) -> Gain21/1
  Constant8/1 -> Switch7/1
  Switch7/1 -> Consumer Station1/2(V_12)
  [v12_31] -> Switch7/3
  From16/1 -> Switch7/2
  Signal Specification6/1 -> [q_30_v3]
  [v11_30] -> Switch3/3
  Signal Specification1/1 -> [tank_30_mm]
  Switch5/1 -> Consumer Station/2(V_12)
  [v12_30] -> Switch5/3
  Signal Specification2/1 -> [tank_31_mm]
  Signal Specification17/1 -> [p12_31]
  Gain2/1 -> Signal Specification2/1
  Consumer Station2/2(P_12) -> Gain20/1
  Gain1/1 -> Signal Specification1/1
  From3/1 -> Switch4/2
  Constant/1 -> Consumer Station/5(V_22), Consumer Station/4(V_21)
  Gain21/1 -> Signal Specification21/1
  Constant4/1 -> Switch5/1
  Consumer Station/3(P_13) -> Gain15/1
  Consumer Station/19(Q1_13) -> Gain6/1
  Constant6/1 -> Consumer Station2/5(V_22), Consumer Station2/4(V_21)
  Constant2/1 -> Switch3/1
  Signal Specification20/1 -> [p12_32]
  From14/1 -> Switch5/2
  From1/1 -> Switch1/2
  Signal Specification21/1 -> [p13_32]
  Gain10/1 -> Signal Specification10/1
  Signal Specification9/1 -> [q_31_v3]
  Signal Specification22/1 -> [q_34_v1]
  [v12_34] -> Switch12/3
  Gain24/1 -> Signal Specification24/1
  Consumer Station3/17(Q1_11) -> Gain22/1
  From22/1 -> Switch10/2
  Consumer Station3/1(P_11) -> Gain25/1
  Signal Specification26/1 -> [p12_34]
  [bottom_valve_34] -> Switch10/3
  Signal Specification27/1 -> [p13_34]
  Gain25/1 -> Signal Specification25/1
  Consumer Station3/2(P_12) -> Gain26/1
  Signal Specification28/1 -> [tank_34_mm]
  Gain22/1 -> Signal Specification22/1
  Gain27/1 -> Signal Specification27/1
  Signal Specification23/1 -> [q_34_v2]
  Constant15/1 -> Switch11/1
  Consumer Station3/18(Q1_12) -> Gain23/1
  Constant13/1 -> Consumer Station3/5(V_22), Consumer Station3/4(V_21)
  Constant12/1 -> Switch12/1
  Gain23/1 -> Signal Specification23/1
  Gain26/1 -> Signal Specification26/1
  Switch11/1 -> Consumer Station3/1(V_11)
  Switch12/1 -> Consumer Station3/2(V_12)
  Consumer Station3/3(P_13) -> Gain27/1
  [v11_34] -> Switch11/3
  Constant14/1 -> Switch10/1
  Consumer Station3/8(dP_2) -> Gain28/1
  Signal Specification24/1 -> [q_34_v3]
  Switch10/1 -> Consumer Station3/3(V_13)
  From21/1 -> Switch12/2
  Signal Specification25/1 -> [p11_34]
  From20/1 -> Switch11/2
  Gain28/1 -> Signal Specification28/1
  Consumer Station3/19(Q1_13) -> Gain24/1

== system On_off_1_pumpstation/ /Piping -1 ==
  note: Free
  Constant : Constant  Value=zeros(19,1)
  Demux : Demux  Outputs=[4 12 8]
  Demux1 : Demux
  Demux2 : Demux  Outputs=12
  Demux3 : Demux
  Modbus Read : modbusMatLib/Modbus Read  registry=0  ipAddress='192.168.100.20'  port=502
  Modbus Write : modbusMatLib/Modbus Write  registry=001  port=502  ipAddress='192.168.100.20'
  Q3_1 : Outport  VectorParamsAs1DForOutWhenUnconnected=off
  Q3_2 : Outport  Port=2  VectorParamsAs1DForOutWhenUnconnected=off
  Q3_3 : Outport  Port=3  VectorParamsAs1DForOutWhenUnconnected=off
  Q3_4 : Outport  Port=4  VectorParamsAs1DForOutWhenUnconnected=off
  P_11 : Outport  Port=5  VectorParamsAs1DForOutWhenUnconnected=off
  P_12 : Outport  Port=6  VectorParamsAs1DForOutWhenUnconnected=off
  P_13 : Outport  Port=7  VectorParamsAs1DForOutWhenUnconnected=off
  P_21 : Outport  Port=8  VectorParamsAs1DForOutWhenUnconnected=off
  P_22 : Outport  Port=9  VectorParamsAs1DForOutWhenUnconnected=off
  P_23 : Outport  Port=10  VectorParamsAs1DForOutWhenUnconnected=off
  P_31 : Outport  Port=11  VectorParamsAs1DForOutWhenUnconnected=off
  P_32 : Outport  Port=12  VectorParamsAs1DForOutWhenUnconnected=off
  P_33 : Outport  Port=13  VectorParamsAs1DForOutWhenUnconnected=off
  P_41 : Outport  Port=14  VectorParamsAs1DForOutWhenUnconnected=off
  P_42 : Outport  Port=15  VectorParamsAs1DForOutWhenUnconnected=off
  P_43 : Outport  Port=16  VectorParamsAs1DForOutWhenUnconnected=off
  wires:
  Demux1/4 -> Q3_4/1
  Demux1/2 -> Q3_2/1
  Demux1/1 -> Q3_1/1
  Demux1/3 -> Q3_3/1
  Demux/1 -> Demux1/1
  Modbus Read/1 -> Demux/1
  Constant/1 -> Modbus Write/1
  Demux/2 -> Demux2/1
  Demux/3 -> Demux3/1
  Demux2/1 -> P_11/1
  Demux2/2 -> P_12/1
  Demux2/3 -> P_13/1
  Demux2/4 -> P_21/1
  Demux2/5 -> P_22/1
  Demux2/6 -> P_23/1
  Demux2/7 -> P_31/1
  Demux2/8 -> P_32/1
  Demux2/9 -> P_33/1
  Demux2/10 -> P_41/1
  Demux2/11 -> P_42/1
  Demux2/12 -> P_43/1

== system On_off_1_pumpstation/ /Piping -2 ==
  note: Free
  Constant : Constant  Value=zeros(19,1)
  Demux : Demux  Outputs=[4 12 8]
  Demux1 : Demux
  Demux2 : Demux  Outputs=12
  Demux3 : Demux
  Modbus Read : modbusMatLib/Modbus Read  registry=0  ipAddress='192.168.100.21'  port=502
  Modbus Write : modbusMatLib/Modbus Write  registry=001  port=502  ipAddress='192.168.100.21'
  Q3_1 : Outport  VectorParamsAs1DForOutWhenUnconnected=off
  Q3_2 : Outport  Port=2  VectorParamsAs1DForOutWhenUnconnected=off
  Q3_3 : Outport  Port=3  VectorParamsAs1DForOutWhenUnconnected=off
  Q3_4 : Outport  Port=4  VectorParamsAs1DForOutWhenUnconnected=off
  P_11 : Outport  Port=5  VectorParamsAs1DForOutWhenUnconnected=off
  P_12 : Outport  Port=6  VectorParamsAs1DForOutWhenUnconnected=off
  P_13 : Outport  Port=7  VectorParamsAs1DForOutWhenUnconnected=off
  P_21 : Outport  Port=8  VectorParamsAs1DForOutWhenUnconnected=off
  P_22 : Outport  Port=9  VectorParamsAs1DForOutWhenUnconnected=off
  P_23 : Outport  Port=10  VectorParamsAs1DForOutWhenUnconnected=off
  P_31 : Outport  Port=11  VectorParamsAs1DForOutWhenUnconnected=off
  P_32 : Outport  Port=12  VectorParamsAs1DForOutWhenUnconnected=off
  P_33 : Outport  Port=13  VectorParamsAs1DForOutWhenUnconnected=off
  P_41 : Outport  Port=14  VectorParamsAs1DForOutWhenUnconnected=off
  P_42 : Outport  Port=15  VectorParamsAs1DForOutWhenUnconnected=off
  P_43 : Outport  Port=16  VectorParamsAs1DForOutWhenUnconnected=off
  wires:
  Demux1/4 -> Q3_4/1
  Demux1/2 -> Q3_2/1
  Demux1/1 -> Q3_1/1
  Demux1/3 -> Q3_3/1
  Demux/1 -> Demux1/1
  Modbus Read/1 -> Demux/1
  Constant/1 -> Modbus Write/1
  Demux/2 -> Demux2/1
  Demux/3 -> Demux3/1
  Demux2/1 -> P_11/1
  Demux2/2 -> P_12/1
  Demux2/3 -> P_13/1
  Demux2/4 -> P_21/1
  Demux2/5 -> P_22/1
  Demux2/6 -> P_23/1
  Demux2/7 -> P_31/1
  Demux2/8 -> P_32/1
  Demux2/9 -> P_33/1
  Demux2/10 -> P_41/1
  Demux2/11 -> P_42/1
  Demux2/12 -> P_43/1

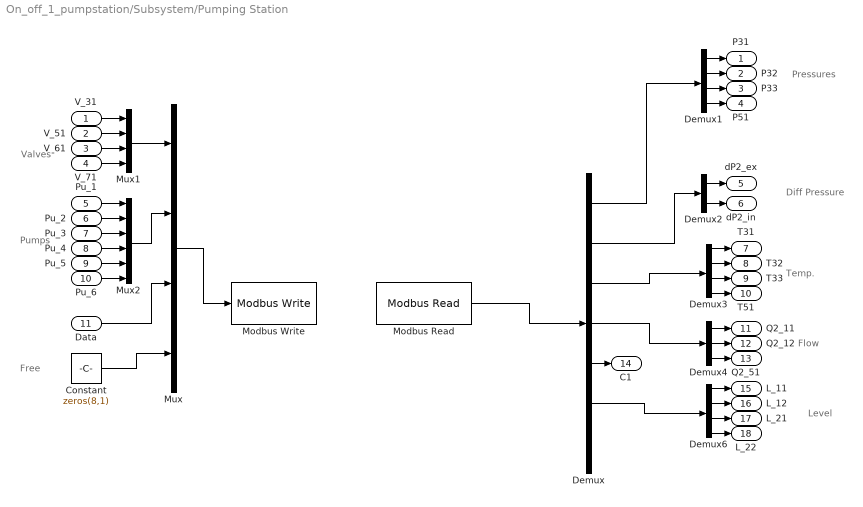
== system On_off_1_pumpstation/Subsystem/Pumping Station ==
  note: Free
  note: Pumps
  note: Valves
  note: Flow
  note: Temp.
  note: Diff Pressure
  note: Pressures
  note: Level
  V_31 : Inport
  V_51 : Inport  Port=2
  V_61 : Inport  Port=3
  V_71 : Inport  Port=4
  Pu_1 : Inport  Port=5
  Pu_2 : Inport  Port=6
  Pu_3 : Inport  Port=7
  Pu_4 : Inport  Port=8
  Pu_5 : Inport  Port=9
  Pu_6 : Inport  Port=10
  Data : Inport  Port=11
  Constant : Constant  Value=zeros(8,1)
  Demux : Demux  Outputs=[4 2 4 3 1 4 6]
  Demux1 : Demux
  Demux2 : Demux  Outputs=2
  Demux3 : Demux
  Demux4 : Demux  Outputs=3
  Demux6 : Demux
  Modbus Read : modbusMatLib/Modbus Read  registry=0  ipAddress='192.168.100.144'  port=502
  Modbus Write : modbusMatLib/Modbus Write  registry=001  port=502  ipAddress='192.168.100.144'
  Mux : Mux
  Mux1 : Mux
  Mux2 : Mux  Inputs=6
  P31 : Outport  VectorParamsAs1DForOutWhenUnconnected=off
  P32 : Outport  Port=2  VectorParamsAs1DForOutWhenUnconnected=off
  P33 : Outport  Port=3  VectorParamsAs1DForOutWhenUnconnected=off
  P51 : Outport  Port=4  VectorParamsAs1DForOutWhenUnconnected=off
  dP2_ex : Outport  Port=5  VectorParamsAs1DForOutWhenUnconnected=off
  dP2_in : Outport  Port=6  VectorParamsAs1DForOutWhenUnconnected=off
  T31 : Outport  Port=7  VectorParamsAs1DForOutWhenUnconnected=off
  T32 : Outport  Port=8  VectorParamsAs1DForOutWhenUnconnected=off
  T33 : Outport  Port=9  VectorParamsAs1DForOutWhenUnconnected=off
  T51 : Outport  Port=10  VectorParamsAs1DForOutWhenUnconnected=off
  Q2_11 : Outport  Port=11  VectorParamsAs1DForOutWhenUnconnected=off
  Q2_12 : Outport  Port=12  VectorParamsAs1DForOutWhenUnconnected=off
  Q2_51 : Outport  Port=13  VectorParamsAs1DForOutWhenUnconnected=off
  C1 : Outport  Port=14  VectorParamsAs1DForOutWhenUnconnected=off
  L_11 : Outport  Port=15  VectorParamsAs1DForOutWhenUnconnected=off
  L_12 : Outport  Port=16  VectorParamsAs1DForOutWhenUnconnected=off
  L_21 : Outport  Port=17  VectorParamsAs1DForOutWhenUnconnected=off
  L_22 : Outport  Port=18  VectorParamsAs1DForOutWhenUnconnected=off
  wires:
  Demux4/1 -> Q2_11/1
  Demux/2 -> Demux2/1
  Demux/4 -> Demux4/1
  Demux2/1 -> dP2_ex/1
  Demux/3 -> Demux3/1
  Demux/6 -> Demux6/1
  Demux/1 -> Demux1/1
  Demux3/4 -> T51/1
  Demux1/4 -> P51/1
  Demux3/2 -> T32/1
  Modbus Read/1 -> Demux/1
  Demux6/1 -> L_11/1
  Demux6/2 -> L_12/1
  Demux4/3 -> Q2_51/1
  Demux4/2 -> Q2_12/1
  Demux6/3 -> L_21/1
  Demux6/4 -> L_22/1
  Demux3/3 -> T33/1
  Demux1/1 -> P31/1
  Demux1/2 -> P32/1
  Demux/5 -> C1/1
  Demux1/3 -> P33/1
  Demux2/2 -> dP2_in/1
  Demux3/1 -> T31/1
  Mux/1 -> Modbus Write/1
  Mux1/1 -> Mux/1
  V_31/1 -> Mux1/1
  V_51/1 -> Mux1/2
  V_61/1 -> Mux1/3
  V_71/1 -> Mux1/4
  Pu_4/1 -> Mux2/4
  Pu_3/1 -> Mux2/3
  Pu_1/1 -> Mux2/1
  Pu_2/1 -> Mux2/2
  Mux2/1 -> Mux/2
  Pu_5/1 -> Mux2/5
  Pu_6/1 -> Mux2/6
  Data/1 -> Mux/3
  Constant/1 -> Mux/4

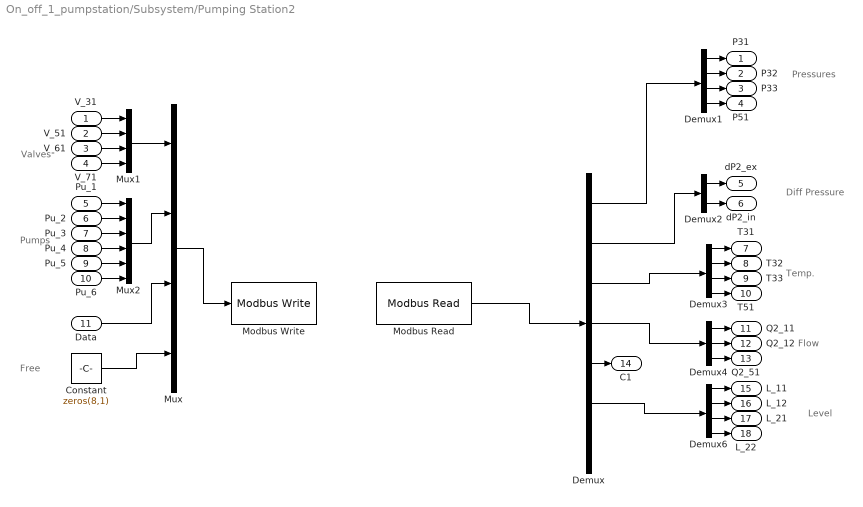
== system On_off_1_pumpstation/Subsystem/Pumping Station2 ==
  note: Free
  note: Pumps
  note: Valves
  note: Flow
  note: Temp.
  note: Diff Pressure
  note: Pressures
  note: Level
  V_31 : Inport
  V_51 : Inport  Port=2
  V_61 : Inport  Port=3
  V_71 : Inport  Port=4
  Pu_1 : Inport  Port=5
  Pu_2 : Inport  Port=6
  Pu_3 : Inport  Port=7
  Pu_4 : Inport  Port=8
  Pu_5 : Inport  Port=9
  Pu_6 : Inport  Port=10
  Data : Inport  Port=11
  Constant : Constant  Value=zeros(8,1)
  Demux : Demux  Outputs=[4 2 4 3 1 4 6]
  Demux1 : Demux
  Demux2 : Demux  Outputs=2
  Demux3 : Demux
  Demux4 : Demux  Outputs=3
  Demux6 : Demux
  Modbus Read : modbusMatLib/Modbus Read  registry=0  ipAddress='192.168.100.41'  port=502
  Modbus Write : modbusMatLib/Modbus Write  registry=001  port=502  ipAddress='192.168.100.41'
  Mux : Mux
  Mux1 : Mux
  Mux2 : Mux  Inputs=6
  P31 : Outport  VectorParamsAs1DForOutWhenUnconnected=off
  P32 : Outport  Port=2  VectorParamsAs1DForOutWhenUnconnected=off
  P33 : Outport  Port=3  VectorParamsAs1DForOutWhenUnconnected=off
  P51 : Outport  Port=4  VectorParamsAs1DForOutWhenUnconnected=off
  dP2_ex : Outport  Port=5  VectorParamsAs1DForOutWhenUnconnected=off
  dP2_in : Outport  Port=6  VectorParamsAs1DForOutWhenUnconnected=off
  T31 : Outport  Port=7  VectorParamsAs1DForOutWhenUnconnected=off
  T32 : Outport  Port=8  VectorParamsAs1DForOutWhenUnconnected=off
  T33 : Outport  Port=9  VectorParamsAs1DForOutWhenUnconnected=off
  T51 : Outport  Port=10  VectorParamsAs1DForOutWhenUnconnected=off
  Q2_11 : Outport  Port=11  VectorParamsAs1DForOutWhenUnconnected=off
  Q2_12 : Outport  Port=12  VectorParamsAs1DForOutWhenUnconnected=off
  Q2_51 : Outport  Port=13  VectorParamsAs1DForOutWhenUnconnected=off
  C1 : Outport  Port=14  VectorParamsAs1DForOutWhenUnconnected=off
  L_11 : Outport  Port=15  VectorParamsAs1DForOutWhenUnconnected=off
  L_12 : Outport  Port=16  VectorParamsAs1DForOutWhenUnconnected=off
  L_21 : Outport  Port=17  VectorParamsAs1DForOutWhenUnconnected=off
  L_22 : Outport  Port=18  VectorParamsAs1DForOutWhenUnconnected=off
  wires:
  Demux4/1 -> Q2_11/1
  Demux/2 -> Demux2/1
  Demux/4 -> Demux4/1
  Demux2/1 -> dP2_ex/1
  Demux/3 -> Demux3/1
  Demux/6 -> Demux6/1
  Demux/1 -> Demux1/1
  Demux3/4 -> T51/1
  Demux1/4 -> P51/1
  Demux3/2 -> T32/1
  Modbus Read/1 -> Demux/1
  Demux6/1 -> L_11/1
  Demux6/2 -> L_12/1
  Demux4/3 -> Q2_51/1
  Demux4/2 -> Q2_12/1
  Demux6/3 -> L_21/1
  Demux6/4 -> L_22/1
  Demux3/3 -> T33/1
  Demux1/1 -> P31/1
  Demux1/2 -> P32/1
  Demux/5 -> C1/1
  Demux1/3 -> P33/1
  Demux2/2 -> dP2_in/1
  Demux3/1 -> T31/1
  Mux/1 -> Modbus Write/1
  Mux1/1 -> Mux/1
  V_31/1 -> Mux1/1
  V_51/1 -> Mux1/2
  V_61/1 -> Mux1/3
  V_71/1 -> Mux1/4
  Pu_4/1 -> Mux2/4
  Pu_3/1 -> Mux2/3
  Pu_1/1 -> Mux2/1
  Pu_2/1 -> Mux2/2
  Mux2/1 -> Mux/2
  Pu_5/1 -> Mux2/5
  Pu_6/1 -> Mux2/6
  Data/1 -> Mux/3
  Constant/1 -> Mux/4

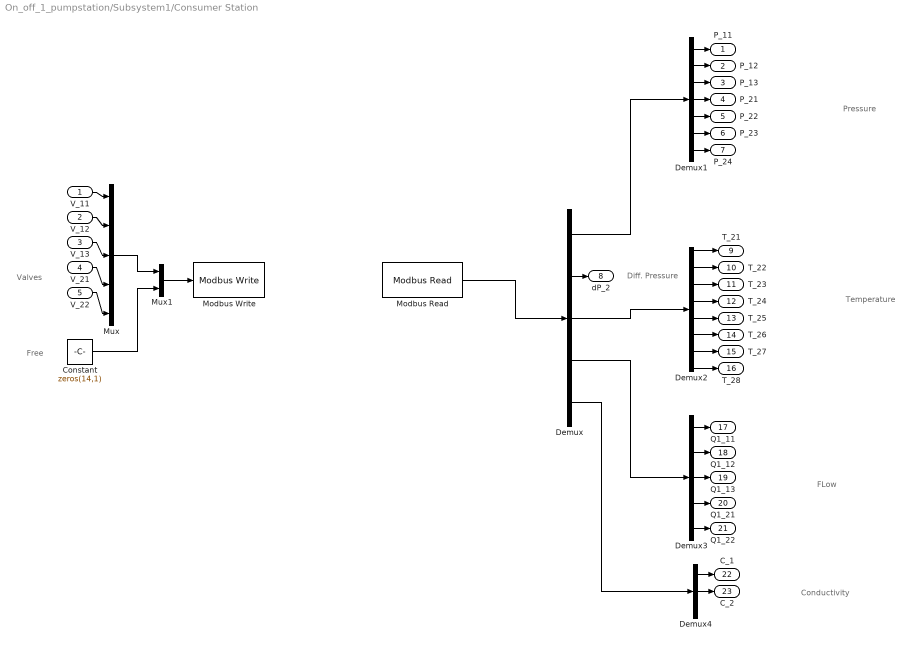
== system On_off_1_pumpstation/Subsystem1/Consumer Station ==
  note: Pressure
  note: Temperature
  note: FLow
  note: Conductivity
  note: Valves
  note: Diff. Pressure
  note: Free
  V_11 : Inport
  V_12 : Inport  Port=2
  V_13 : Inport  Port=3
  V_21 : Inport  Port=4
  V_22 : Inport  Port=5
  Constant : Constant  Value=zeros(14,1)
  Demux : Demux  Outputs=[7 1 8 5 3]
  Demux1 : Demux  Outputs=7
  Demux2 : Demux  Outputs=8
  Demux3 : Demux  Outputs=5
  Demux4 : Demux  Outputs=3
  Modbus Read : modbusMatLib/Modbus Read  registry=0  ipAddress='192.168.100.30'  port=502
  Modbus Write : modbusMatLib/Modbus Write  registry=001  port=502  ipAddress='192.168.100.30'
  Mux : Mux  Inputs=5
  Mux1 : Mux  Inputs=2
  P_11 : Outport  VectorParamsAs1DForOutWhenUnconnected=off
  P_12 : Outport  Port=2  VectorParamsAs1DForOutWhenUnconnected=off
  P_13 : Outport  Port=3  VectorParamsAs1DForOutWhenUnconnected=off
  P_21 : Outport  Port=4  VectorParamsAs1DForOutWhenUnconnected=off
  P_22 : Outport  Port=5  VectorParamsAs1DForOutWhenUnconnected=off
  P_23 : Outport  Port=6  VectorParamsAs1DForOutWhenUnconnected=off
  P_24 : Outport  Port=7  VectorParamsAs1DForOutWhenUnconnected=off
  dP_2 : Outport  Port=8  VectorParamsAs1DForOutWhenUnconnected=off
  T_21 : Outport  Port=9  VectorParamsAs1DForOutWhenUnconnected=off
  T_22 : Outport  Port=10  VectorParamsAs1DForOutWhenUnconnected=off
  T_23 : Outport  Port=11  VectorParamsAs1DForOutWhenUnconnected=off
  T_24 : Outport  Port=12  VectorParamsAs1DForOutWhenUnconnected=off
  T_25 : Outport  Port=13  VectorParamsAs1DForOutWhenUnconnected=off
  T_26 : Outport  Port=14  VectorParamsAs1DForOutWhenUnconnected=off
  T_27 : Outport  Port=15  VectorParamsAs1DForOutWhenUnconnected=off
  T_28 : Outport  Port=16  VectorParamsAs1DForOutWhenUnconnected=off
  Q1_11 : Outport  Port=17  VectorParamsAs1DForOutWhenUnconnected=off
  Q1_12 : Outport  Port=18  VectorParamsAs1DForOutWhenUnconnected=off
  Q1_13 : Outport  Port=19  VectorParamsAs1DForOutWhenUnconnected=off
  Q1_21 : Outport  Port=20  VectorParamsAs1DForOutWhenUnconnected=off
  Q1_22 : Outport  Port=21  VectorParamsAs1DForOutWhenUnconnected=off
  C_1 : Outport  Port=22  VectorParamsAs1DForOutWhenUnconnected=off
  C_2 : Outport  Port=23  VectorParamsAs1DForOutWhenUnconnected=off
  wires:
  Mux/1 -> Mux1/1
  Mux1/1 -> Modbus Write/1
  Constant/1 -> Mux1/2
  Demux1/5 -> P_22/1
  V_12/1 -> Mux/2
  Demux1/6 -> P_23/1
  Demux1/3 -> P_13/1
  Demux1/4 -> P_21/1
  V_13/1 -> Mux/3
  Demux3/2 -> Q1_12/1
  Demux3/5 -> Q1_22/1
  Demux/2 -> dP_2/1
  Demux3/1 -> Q1_11/1
  Demux1/2 -> P_12/1
  Demux2/5 -> T_25/1
  Demux4/1 -> C_1/1
  V_21/1 -> Mux/4
  Demux3/3 -> Q1_13/1
  Demux1/1 -> P_11/1
  Demux3/4 -> Q1_21/1
  V_11/1 -> Mux/1
  Demux2/4 -> T_24/1
  Demux2/3 -> T_23/1
  Demux2/2 -> T_22/1
  Demux2/1 -> T_21/1
  Demux1/7 -> P_24/1
  V_22/1 -> Mux/5
  Demux2/7 -> T_27/1
  Demux/5 -> Demux4/1
  Demux/1 -> Demux1/1
  Demux2/8 -> T_28/1
  Demux4/2 -> C_2/1
  Demux/3 -> Demux2/1
  Demux/4 -> Demux3/1
  Modbus Read/1 -> Demux/1
  Demux2/6 -> T_26/1

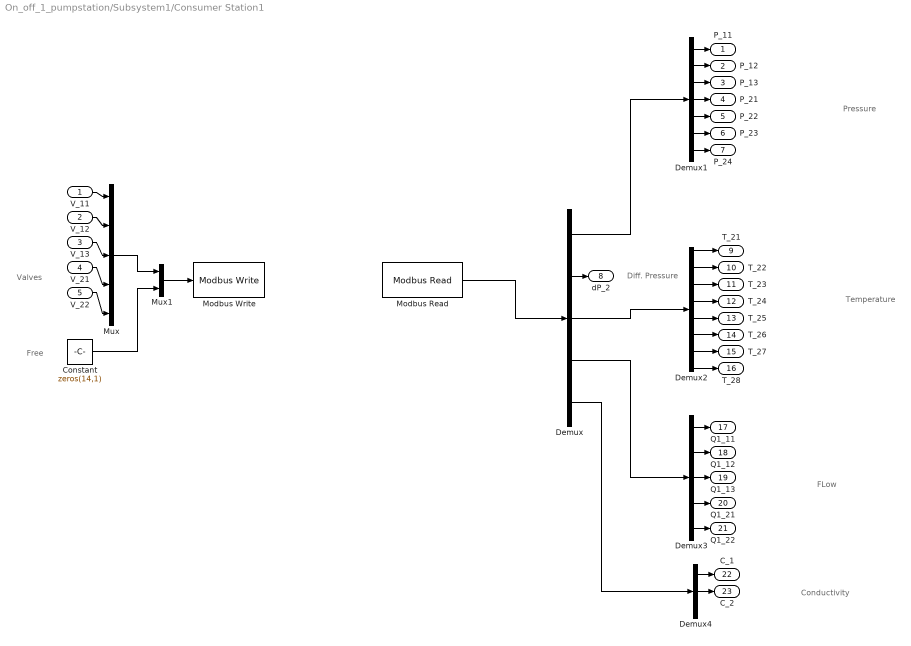
== system On_off_1_pumpstation/Subsystem1/Consumer Station1 ==
  note: Pressure
  note: Temperature
  note: FLow
  note: Conductivity
  note: Valves
  note: Diff. Pressure
  note: Free
  V_11 : Inport
  V_12 : Inport  Port=2
  V_13 : Inport  Port=3
  V_21 : Inport  Port=4
  V_22 : Inport  Port=5
  Constant : Constant  Value=zeros(14,1)
  Demux : Demux  Outputs=[7 1 8 5 3]
  Demux1 : Demux  Outputs=7
  Demux2 : Demux  Outputs=8
  Demux3 : Demux  Outputs=5
  Demux4 : Demux  Outputs=3
  Modbus Read : modbusMatLib/Modbus Read  registry=0  ipAddress='192.168.100.31'  port=502
  Modbus Write : modbusMatLib/Modbus Write  registry=001  port=502  ipAddress='192.168.100.31'
  Mux : Mux  Inputs=5
  Mux1 : Mux  Inputs=2
  P_11 : Outport  VectorParamsAs1DForOutWhenUnconnected=off
  P_12 : Outport  Port=2  VectorParamsAs1DForOutWhenUnconnected=off
  P_13 : Outport  Port=3  VectorParamsAs1DForOutWhenUnconnected=off
  P_21 : Outport  Port=4  VectorParamsAs1DForOutWhenUnconnected=off
  P_22 : Outport  Port=5  VectorParamsAs1DForOutWhenUnconnected=off
  P_23 : Outport  Port=6  VectorParamsAs1DForOutWhenUnconnected=off
  P_24 : Outport  Port=7  VectorParamsAs1DForOutWhenUnconnected=off
  dP_2 : Outport  Port=8  VectorParamsAs1DForOutWhenUnconnected=off
  T_21 : Outport  Port=9  VectorParamsAs1DForOutWhenUnconnected=off
  T_22 : Outport  Port=10  VectorParamsAs1DForOutWhenUnconnected=off
  T_23 : Outport  Port=11  VectorParamsAs1DForOutWhenUnconnected=off
  T_24 : Outport  Port=12  VectorParamsAs1DForOutWhenUnconnected=off
  T_25 : Outport  Port=13  VectorParamsAs1DForOutWhenUnconnected=off
  T_26 : Outport  Port=14  VectorParamsAs1DForOutWhenUnconnected=off
  T_27 : Outport  Port=15  VectorParamsAs1DForOutWhenUnconnected=off
  T_28 : Outport  Port=16  VectorParamsAs1DForOutWhenUnconnected=off
  Q1_11 : Outport  Port=17  VectorParamsAs1DForOutWhenUnconnected=off
  Q1_12 : Outport  Port=18  VectorParamsAs1DForOutWhenUnconnected=off
  Q1_13 : Outport  Port=19  VectorParamsAs1DForOutWhenUnconnected=off
  Q1_21 : Outport  Port=20  VectorParamsAs1DForOutWhenUnconnected=off
  Q1_22 : Outport  Port=21  VectorParamsAs1DForOutWhenUnconnected=off
  C_1 : Outport  Port=22  VectorParamsAs1DForOutWhenUnconnected=off
  C_2 : Outport  Port=23  VectorParamsAs1DForOutWhenUnconnected=off
  wires:
  Mux/1 -> Mux1/1
  Mux1/1 -> Modbus Write/1
  Constant/1 -> Mux1/2
  Demux1/5 -> P_22/1
  V_12/1 -> Mux/2
  Demux1/6 -> P_23/1
  Demux1/3 -> P_13/1
  Demux1/4 -> P_21/1
  V_13/1 -> Mux/3
  Demux3/2 -> Q1_12/1
  Demux3/5 -> Q1_22/1
  Demux/2 -> dP_2/1
  Demux3/1 -> Q1_11/1
  Demux1/2 -> P_12/1
  Demux2/5 -> T_25/1
  Demux4/1 -> C_1/1
  V_21/1 -> Mux/4
  Demux3/3 -> Q1_13/1
  Demux1/1 -> P_11/1
  Demux3/4 -> Q1_21/1
  V_11/1 -> Mux/1
  Demux2/4 -> T_24/1
  Demux2/3 -> T_23/1
  Demux2/2 -> T_22/1
  Demux2/1 -> T_21/1
  Demux1/7 -> P_24/1
  V_22/1 -> Mux/5
  Demux2/7 -> T_27/1
  Demux/5 -> Demux4/1
  Demux/1 -> Demux1/1
  Demux2/8 -> T_28/1
  Demux4/2 -> C_2/1
  Demux/3 -> Demux2/1
  Demux/4 -> Demux3/1
  Modbus Read/1 -> Demux/1
  Demux2/6 -> T_26/1
